simulink model "DC_Motor_Mathematical_Modelling"  (R2015a)
settings: Solver=ode45  StartTime=0.0  StopTime=2  RelTol=1e-3
values from neighbouring files (symbols this model uses):
  B = 0.01    [DC_Motor_Mathematical_Modelling_Script.m]
  J = 0.5    [DC_Motor_Mathematical_Modelling_Script.m]
  K = 1.25    [DC_Motor_Mathematical_Modelling_Script.m]
  L = 0.05    [DC_Motor_Mathematical_Modelling_Script.m]
  R = 0.4    [DC_Motor_Mathematical_Modelling_Script.m]
settings Model: Creator=Koustubh  LastModifiedBy=Koustubh

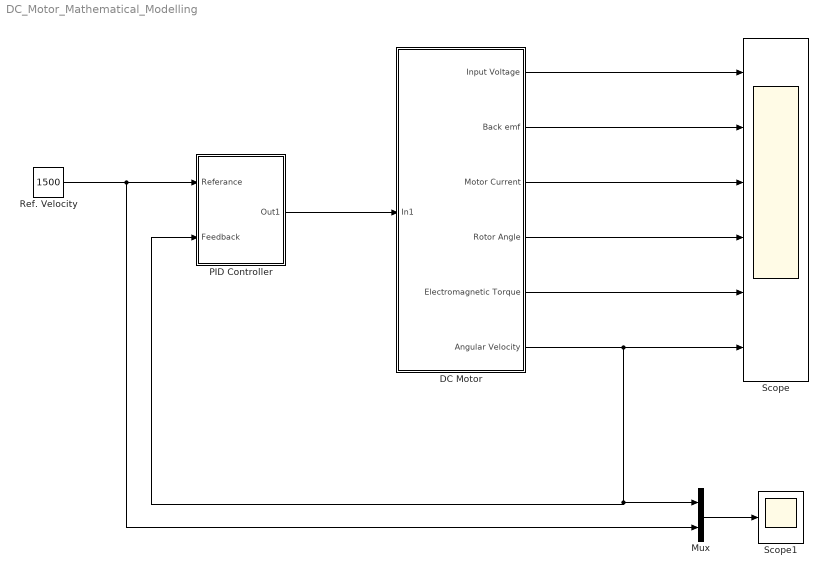
== system DC_Motor_Mathematical_Modelling ==
  DC Motor : Subsystem
  Mux : Mux  Inputs=2
  PID Controller : Subsystem
  Ref. Velocity : Constant  Value=1500
  Scope : Scope  NumInputPorts=6
      settings: YMin=-5~-5~-5~-5~-5~-5  YMax=5~5~5~5~5~5
  Scope1 : Scope
  wires:
  Ref. Velocity/1 -> Mux/2, PID Controller/1(Referance)
  PID Controller/1(Out1) -> DC Motor/1(In1)
  DC Motor/1(Input Voltage) -> Scope/1
  DC Motor/2(Back emf) -> Scope/2
  DC Motor/3(Motor Current) -> Scope/3
  DC Motor/4(Rotor Angle) -> Scope/4
  DC Motor/5(Electromagnetic Torque) -> Scope/5
  DC Motor/6(Angular Velocity) -> Mux/1, PID Controller/2(Feedback), Scope/6
  Mux/1 -> Scope1/1

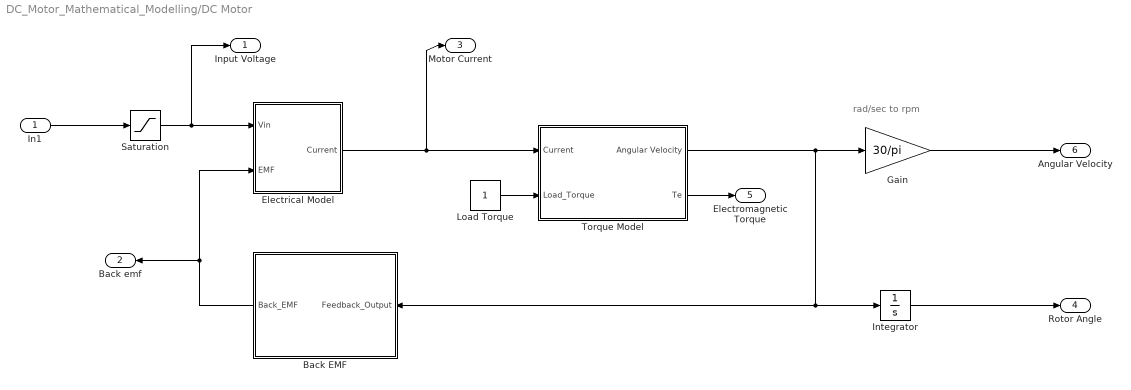
== system DC_Motor_Mathematical_Modelling/DC Motor ==
  note: rad/sec to rpm
  In1 : Inport
  Back EMF : Subsystem
  Electrical Model : Subsystem
  Gain : Gain  Gain=30/pi
  Integrator : Integrator
  Load Torque : Constant
  Saturation : Saturate  UpperLimit=200  LowerLimit=-200
  Torque Model : Subsystem
  Input Voltage : Outport
  Back emf : Outport  Port=2
  Motor Current : Outport  Port=3
  Rotor Angle : Outport  Port=4
  Electromagnetic Torque : Outport  Port=5
  Angular Velocity : Outport  Port=6
  wires:
  In1/1 -> Saturation/1
  Saturation/1 -> Input Voltage/1, Electrical Model/1(Vin)
  Back EMF/1(Back_EMF) -> Back emf/1, Electrical Model/2(EMF)
  Load Torque/1 -> Torque Model/2(Load_Torque)
  Electrical Model/1(Current) -> Torque Model/1(Current), Motor Current/1
  Torque Model/1(Angular Velocity) -> Back EMF/1(Feedback_Output), Integrator/1, Gain/1
  Gain/1 -> Angular Velocity/1
  Integrator/1 -> Rotor Angle/1
  Torque Model/2(Te) -> Electromagnetic Torque/1

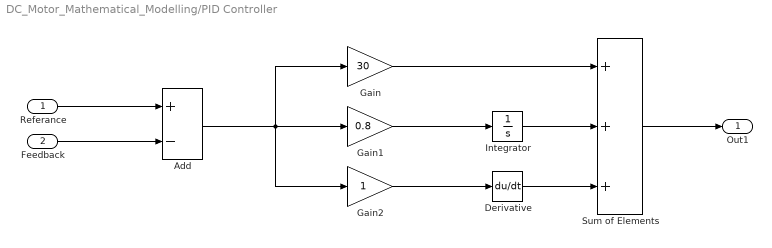
== system DC_Motor_Mathematical_Modelling/PID Controller ==
  Referance : Inport
  Feedback : Inport  Port=2
  Add : Sum  Inputs=+-
  Derivative : Derivative
  Gain : Gain  Gain=30
  Gain1 : Gain  Gain=0.8
  Gain2 : Gain
  Integrator : Integrator
  Sum of Elements : Sum  Inputs=+++
  Out1 : Outport
  wires:
  Referance/1 -> Add/1
  Feedback/1 -> Add/2
  Add/1 -> Gain1/1, Gain2/1, Gain/1
  Gain/1 -> Sum of Elements/1
  Gain2/1 -> Derivative/1
  Derivative/1 -> Sum of Elements/3
  Gain1/1 -> Integrator/1
  Integrator/1 -> Sum of Elements/2
  Sum of Elements/1 -> Out1/1

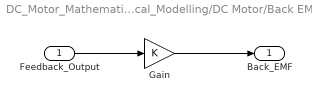
== system DC_Motor_Mathematical_Modelling/DC Motor/Back EMF ==
  Feedback_Output : Inport
  Gain : Gain  Gain=K
  Back_EMF : Outport
  wires:
  Feedback_Output/1 -> Gain/1
  Gain/1 -> Back_EMF/1

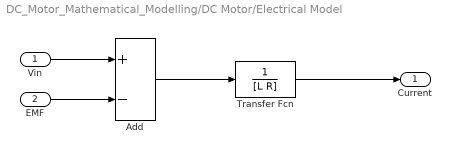
== system DC_Motor_Mathematical_Modelling/DC Motor/Electrical Model ==
  Vin : Inport
  EMF : Inport  Port=2
  Add : Sum  Inputs=+-
  Transfer Fcn : TransferFcn  Denominator=[L R]
  Current : Outport
  wires:
  Add/1 -> Transfer Fcn/1
  EMF/1 -> Add/2
  Vin/1 -> Add/1
  Transfer Fcn/1 -> Current/1

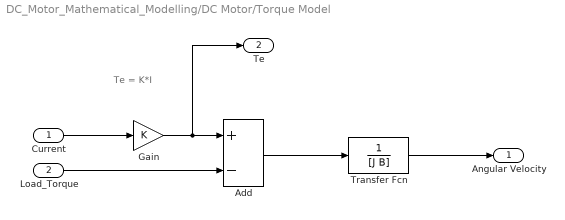
== system DC_Motor_Mathematical_Modelling/DC Motor/Torque Model ==
  note: Te = K*I
  Current : Inport
  Load_Torque : Inport  Port=2
  Add : Sum  Inputs=+-
  Gain : Gain  Gain=K
  Transfer Fcn : TransferFcn  Denominator=[J B]
  Angular Velocity : Outport
  Te : Outport  Port=2
  wires:
  Load_Torque/1 -> Add/2
  Current/1 -> Gain/1
  Gain/1 -> Te/1, Add/1
  Add/1 -> Transfer Fcn/1
  Transfer Fcn/1 -> Angular Velocity/1
